simulink model "Short_Circuit_Test_of_Three_Phase_Transformer"  (R2025a)
settings: Solver=ode23tb  StartTime=0.0  StopTime=0.2  MaxStep=1e-4  RelTol=1e-3
libraries: spsACVoltageSourceLib x3, spsRMSLib x2, spsGroundLib x1, spsPower3phInstantaneousLib x1, spsThreePhaseTransformerTwoWindingsLib x1, spsThreePhaseVIMeasurementLib x1, sps_lib x1
settings Model: Creator=Jawad  LastModifiedBy=Jawad

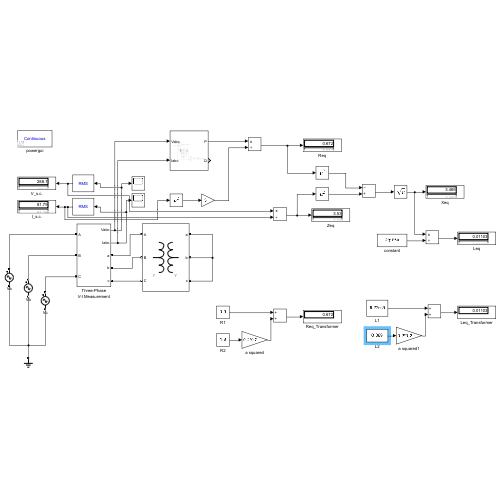
[thumbnail: Simulink's stored preview of the top-level diagram]
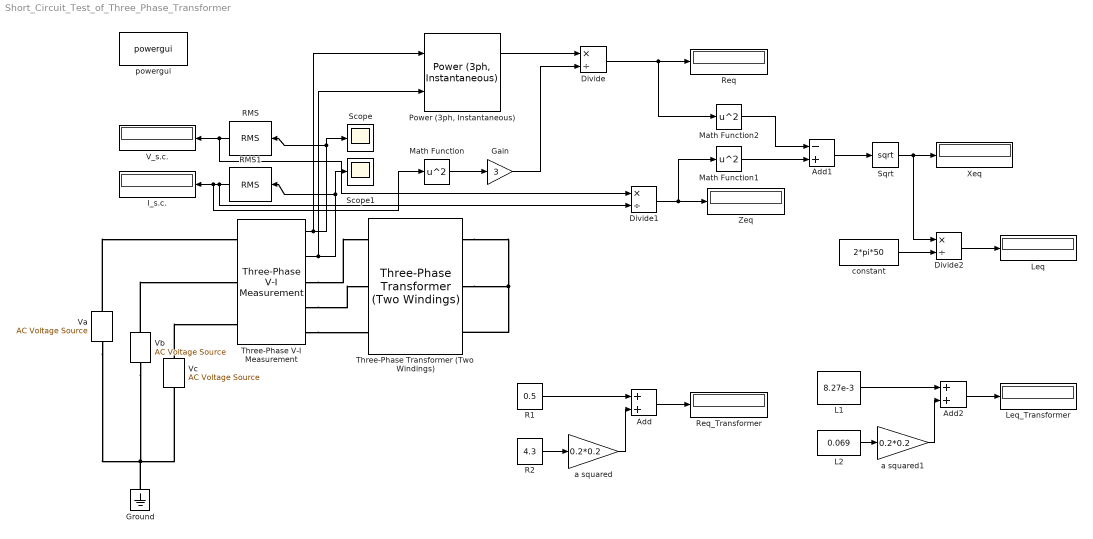
== system Short_Circuit_Test_of_Three_Phase_Transformer ==
  Add : Sum
  Add1 : Sum  Inputs=-+
  Add2 : Sum
  Divide : Product  Inputs=*/
  Divide1 : Product  Inputs=*/
  Divide2 : Product  Inputs=*/
  Gain : Gain  Gain=3
  Ground : spsGroundLib/Ground  LConnTagsString=a
  I_s.c. : Display
  L1 : Constant  Value=8.27e-3
  L2 : Constant  Value=0.069
  Leq : Display
  Leq_Transformer : Display
  Math Function : Math  Operator=square
  Math Function1 : Math  Operator=square
  Math Function2 : Math  Operator=square
  "Power (3ph, Instantaneous)" : spsPower3phInstantaneousLib/Power (3ph, Instantaneous)
  R1 : Constant  Value=0.5
  R2 : Constant  Value=4.3
  RMS : spsRMSLib/RMS  TrueRMS=off  Freq=50  RMSInit=0  Ts=0
  RMS1 : spsRMSLib/RMS  TrueRMS=off  Freq=50  RMSInit=0  Ts=0
  Req : Display
  Req_Transformer : Display
  Scope : Scope
      settings: ActiveDisplayYMinimum=-6736.0902871668777  ActiveDisplayYMaximum=6736.0893810743028
  Scope1 : Scope
  Sqrt : Sqrt
  Three-Phase Transformer (Two Windings) : spsThreePhaseTransformerTwoWindingsLib/Three-Phase Transformer (Two Windings)  Winding1Connection=Y  Winding2Connection=Y  CoreType=Three single-phase transformers  SetSaturation=off  Hysteresis=off  DataFile='hysteresis'  SetInitialFlux=off  Measurements=None  UNITS=SI  NominalPower=[ 2000e3 , 50 ]  Winding1=[6.6e3 0.5 8.27e-3]  Winding2=[33e3 4.3 0.069]  Rm=10000  Lm=500  L0=0.28887  Saturation=[0 0;0.059382 17.153;24.742 21.728]  InitialFluxes=[11.436 -11.436 10.006]  BreakLoop=off  DiscreteSolver=Trapezoidal iterative  DataType=on  TransfoNumber=1
  Three-Phase V-I Measurement : spsThreePhaseVIMeasurementLib/Three-Phase V-I Measurement  VoltageMeasurement=phase-to-ground  SetLabelV=off  LabelV=Vabc  Vpu=off  VpuLL=off  CurrentMeasurement=yes  SetLabelI=off  LabelI=Iabc  Ipu=off  Pbase=100e6  Vbase=500e3  OutputType=Complex  PhasorSimulation=off  PSBequivalent=0
  V_s.c. : Display
  Va : spsACVoltageSourceLib/AC Voltage Source  Amplitude=(0.5e3*sqrt(2))/sqrt(3)  Phase=0  Frequency=50  SampleTime=0  Measurements=None  BusType=swing  Pref=10e3  Qref=0  Qmin=-inf  Qmax=+inf
  Vb : spsACVoltageSourceLib/AC Voltage Source  Amplitude=(0.5e3*sqrt(2))/sqrt(3)  Phase=-120  Frequency=50  SampleTime=0  Measurements=None  BusType=swing  Pref=10e3  Qref=0  Qmin=-inf  Qmax=+inf
  Vc : spsACVoltageSourceLib/AC Voltage Source  Amplitude=(0.5e3*sqrt(2))/sqrt(3)  Phase=120  Frequency=50  SampleTime=0  Measurements=None  BusType=swing  Pref=10e3  Qref=0  Qmin=-inf  Qmax=+inf
  Xeq : Display
  Zeq : Display
  a squared : Gain  Gain=0.2*0.2
  a squared1 : Gain  Gain=0.2*0.2
  constant : Constant  Value=2*pi*50
  powergui : sps_lib/powergui  Priority=1  SimulationMode=Continuous  SampleTime=50e-6  frequency=60  Iterations=50  frequencyindice=50  Pbase=100e6  ErrMax=1e-4  UnitsV=kV  UnitsW=MW  buscounter=0  FunctionMessages=off  echomessages=off  EnableUseOfTLC=off  CurrentSourceSwitches=off  DisableSnubberDevices=off  DisableRonSwitches=off  DisableVfSwitches=off  DisplayEquations=off  AutomaticDiscreteSolvers=off  SolverType=Tustin/Backward Euler (TBE)  Interpol=off  ExternalGateDelay=off  methode=off  Ts=100  x0status=blocks  SPID=on  SwTol=0  HookPort=off  NonlinearTolerance=1e-4  nMaxIteration=100  ContinueOnMaxIteration=off  RestoreLinks=warning  ResistiveCurrentMeasurement=off  Frange=[0:2:500]  Ylog=off  Xlog=on  ShowGrid=off  save=off  variable=ZData  structure=0  ZoomFFT=off  StartTime=0.0  cycles=1  DisplayStyle=1  fundamental=60  FreqAxis=off  MaxFrequency=1000  frequencyindicesteady=1  RmsSteady=1  display=off
  wires:
  Three-Phase V-I Measurement/1 -> "Power (3ph, Instantaneous)"/1, Scope/1, RMS/1
  RMS/1 -> Divide1/1, V_s.c./1
  RMS1/1 -> Divide1/2, Math Function/1, I_s.c./1
  Three-Phase V-I Measurement/2 -> "Power (3ph, Instantaneous)"/2, Scope1/1, RMS1/1
  "Power (3ph, Instantaneous)"/1 -> Divide/1
  Gain/1 -> Divide/2
  Math Function/1 -> Gain/1
  Divide/1 -> Math Function2/1, Req/1
  R1/1 -> Add/1
  R2/1 -> a squared/1
  a squared/1 -> Add/2
  Add/1 -> Req_Transformer/1
  Divide1/1 -> Math Function1/1, Zeq/1
  Math Function1/1 -> Add1/2
  Math Function2/1 -> Add1/1
  Add1/1 -> Sqrt/1
  Sqrt/1 -> Divide2/1, Xeq/1
  constant/1 -> Divide2/2
  Divide2/1 -> Leq/1
  L2/1 -> a squared1/1
  L1/1 -> Add2/1
  Add2/1 -> Leq_Transformer/1
  a squared1/1 -> Add2/2
  connections:
  Vc/LConn1 -- Ground/LConn1 -- Va/LConn1 -- Vb/LConn1
  Vc/RConn1 -- Three-Phase V-I Measurement/LConn3
  Vb/RConn1 -- Three-Phase V-I Measurement/LConn2
  Va/RConn1 -- Three-Phase V-I Measurement/LConn1
  Three-Phase V-I Measurement/RConn3 -- Three-Phase Transformer (Two Windings)/LConn3
  Three-Phase V-I Measurement/RConn1 -- Three-Phase Transformer (Two Windings)/LConn1
  Three-Phase V-I Measurement/RConn2 -- Three-Phase Transformer (Two Windings)/LConn2
  Three-Phase Transformer (Two Windings)/RConn1 -- Three-Phase Transformer (Two Windings)/RConn2 -- Three-Phase Transformer (Two Windings)/RConn3
